simulink model "amr_integrated_delivery_system"  (R2025b)
settings: Solver=FixedStepDiscrete  StartTime=0.0  StopTime=90  FixedStep=0.05  RelTol=1e-3
settings Model: Creator=leeyj  LastModifiedBy=leeyj

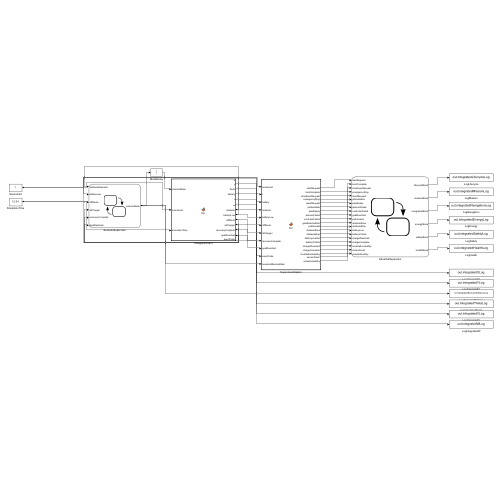
[thumbnail: Simulink's stored preview of the top-level diagram]
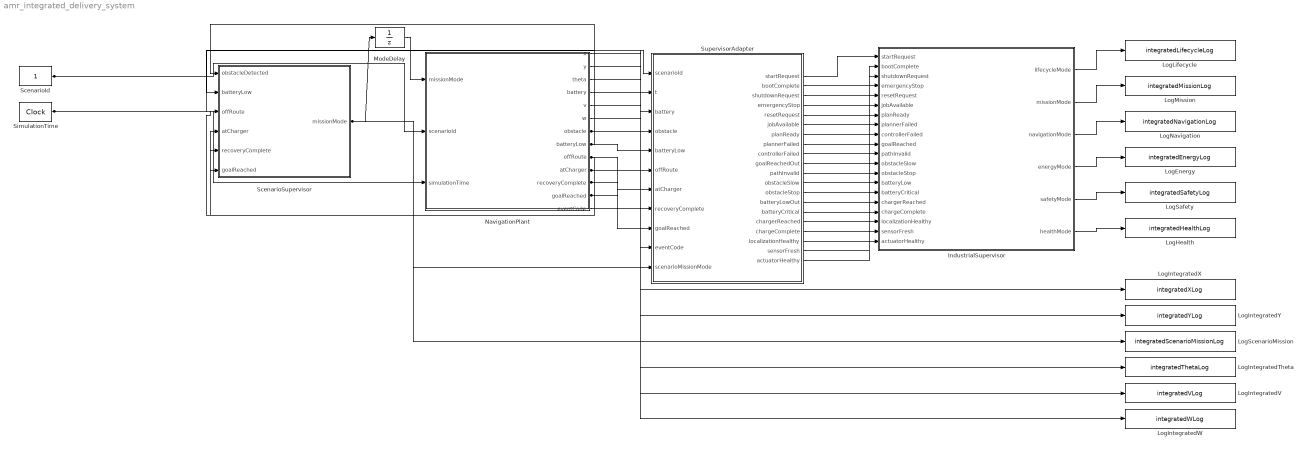
== system amr_integrated_delivery_system ==
  IndustrialSupervisor : Stateflow chart  TreatAsAtomicUnit=on
  LogEnergy : ToWorkspace  VariableName=integratedEnergyLog  SaveFormat=Timeseries  SampleTime=-1
  LogHealth : ToWorkspace  VariableName=integratedHealthLog  SaveFormat=Timeseries  SampleTime=-1
  LogIntegratedTheta : ToWorkspace  VariableName=integratedThetaLog  SaveFormat=Timeseries  SampleTime=-1
  LogIntegratedV : ToWorkspace  VariableName=integratedVLog  SaveFormat=Timeseries  SampleTime=-1
  LogIntegratedW : ToWorkspace  VariableName=integratedWLog  SaveFormat=Timeseries  SampleTime=-1
  LogIntegratedX : ToWorkspace  VariableName=integratedXLog  SaveFormat=Timeseries  SampleTime=-1
  LogIntegratedY : ToWorkspace  VariableName=integratedYLog  SaveFormat=Timeseries  SampleTime=-1
  LogLifecycle : ToWorkspace  VariableName=integratedLifecycleLog  SaveFormat=Timeseries  SampleTime=-1
  LogMission : ToWorkspace  VariableName=integratedMissionLog  SaveFormat=Timeseries  SampleTime=-1
  LogNavigation : ToWorkspace  VariableName=integratedNavigationLog  SaveFormat=Timeseries  SampleTime=-1
  LogSafety : ToWorkspace  VariableName=integratedSafetyLog  SaveFormat=Timeseries  SampleTime=-1
  LogScenarioMission : ToWorkspace  VariableName=integratedScenarioMissionLog  SaveFormat=Timeseries  SampleTime=-1
  ModeDelay : UnitDelay  SampleTime=0.05  HasFrameUpgradeWarning=on
  NavigationPlant : MATLAB Function  TreatAsAtomicUnit=on
  ScenarioId : Constant
  ScenarioSupervisor : Stateflow chart  TreatAsAtomicUnit=on
  SimulationTime : DigitalClock  SampleTime=0.05
  SupervisorAdapter : MATLAB Function  TreatAsAtomicUnit=on
  wires:
  ModeDelay/1 -> NavigationPlant/1(missionMode)
  ScenarioId/1 -> NavigationPlant/2(scenarioId), SupervisorAdapter/1(scenarioId)
  SimulationTime/1 -> NavigationPlant/3(simulationTime), SupervisorAdapter/2(t)
  NavigationPlant/7(obstacle) -> ScenarioSupervisor/1(obstacleDetected), SupervisorAdapter/4(obstacle)
  NavigationPlant/8(batteryLow) -> ScenarioSupervisor/2(batteryLow), SupervisorAdapter/5(batteryLow)
  NavigationPlant/9(offRoute) -> ScenarioSupervisor/3(offRoute), SupervisorAdapter/6(offRoute)
  NavigationPlant/10(atCharger) -> ScenarioSupervisor/4(atCharger), SupervisorAdapter/7(atCharger)
  NavigationPlant/11(recoveryComplete) -> ScenarioSupervisor/5(recoveryComplete), SupervisorAdapter/8(recoveryComplete)
  NavigationPlant/12(goalReached) -> ScenarioSupervisor/6(goalReached), SupervisorAdapter/9(goalReached)
  ScenarioSupervisor/1(missionMode) -> ModeDelay/1, SupervisorAdapter/11(scenarioMissionMode), LogScenarioMission/1
  NavigationPlant/4(battery) -> SupervisorAdapter/3(battery)
  NavigationPlant/13(eventCode) -> SupervisorAdapter/10(eventCode)
  SupervisorAdapter/1(startRequest) -> IndustrialSupervisor/1(startRequest)
  SupervisorAdapter/2(bootComplete) -> IndustrialSupervisor/2(bootComplete)
  SupervisorAdapter/3(shutdownRequest) -> IndustrialSupervisor/3(shutdownRequest)
  SupervisorAdapter/4(emergencyStop) -> IndustrialSupervisor/4(emergencyStop)
  SupervisorAdapter/5(resetRequest) -> IndustrialSupervisor/5(resetRequest)
  SupervisorAdapter/6(jobAvailable) -> IndustrialSupervisor/6(jobAvailable)
  SupervisorAdapter/7(planReady) -> IndustrialSupervisor/7(planReady)
  SupervisorAdapter/8(plannerFailed) -> IndustrialSupervisor/8(plannerFailed)
  SupervisorAdapter/9(controllerFailed) -> IndustrialSupervisor/9(controllerFailed)
  SupervisorAdapter/10(goalReachedOut) -> IndustrialSupervisor/10(goalReached)
  SupervisorAdapter/11(pathInvalid) -> IndustrialSupervisor/11(pathInvalid)
  SupervisorAdapter/12(obstacleSlow) -> IndustrialSupervisor/12(obstacleSlow)
  SupervisorAdapter/13(obstacleStop) -> IndustrialSupervisor/13(obstacleStop)
  SupervisorAdapter/14(batteryLowOut) -> IndustrialSupervisor/14(batteryLow)
  SupervisorAdapter/15(batteryCritical) -> IndustrialSupervisor/15(batteryCritical)
  SupervisorAdapter/16(chargerReached) -> IndustrialSupervisor/16(chargerReached)
  SupervisorAdapter/17(chargeComplete) -> IndustrialSupervisor/17(chargeComplete)
  SupervisorAdapter/18(localizationHealthy) -> IndustrialSupervisor/18(localizationHealthy)
  SupervisorAdapter/19(sensorFresh) -> IndustrialSupervisor/19(sensorFresh)
  SupervisorAdapter/20(actuatorHealthy) -> IndustrialSupervisor/20(actuatorHealthy)
  NavigationPlant/1(x) -> LogIntegratedX/1
  NavigationPlant/2(y) -> LogIntegratedY/1
  IndustrialSupervisor/1(lifecycleMode) -> LogLifecycle/1
  IndustrialSupervisor/2(missionMode) -> LogMission/1
  IndustrialSupervisor/3(navigationMode) -> LogNavigation/1
  IndustrialSupervisor/4(energyMode) -> LogEnergy/1
  IndustrialSupervisor/5(safetyMode) -> LogSafety/1
  IndustrialSupervisor/6(healthMode) -> LogHealth/1
  NavigationPlant/3(theta) -> LogIntegratedTheta/1
  NavigationPlant/5(v) -> LogIntegratedV/1
  NavigationPlant/6(w) -> LogIntegratedW/1

== stateflow chart amr_integrated_delivery_system/IndustrialSupervisor ==
  state Operational
    entry,during:
    lifecycleMode = uint8(2);
    state MissionRegion [parallel]
      settings: executionOrder=1
      state Idle
        entry,during:
        missionMode = uint8(0);
      state AcceptJob
        entry,during:
        missionMode = uint8(1);
      state NavigatePickup
        entry,during:
        missionMode = uint8(2);
      state Loading
        entry,during:
        missionMode = uint8(3);
      state NavigateDropoff
        entry,during:
        missionMode = uint8(4);
      state Unloading
        entry,during:
        missionMode = uint8(5);
      state ReturnHome
        entry,during:
        missionMode = uint8(6);
      (default) -> Idle
      Idle -> AcceptJob : [jobAvailable]
      ReturnHome -> Idle : [goalReached]
      AcceptJob -> NavigatePickup : after(0.5,sec)
      NavigatePickup -> Loading : [goalReached]
      Loading -> NavigateDropoff : after(1,sec)
      NavigateDropoff -> Unloading : [goalReached]
      Unloading -> ReturnHome : after(1,sec)
    state NavigationRegion [parallel]
      settings: executionOrder=2
      state NavIdle
        entry,during:
        navigationMode = uint8(0);
      state Planning
        entry,during:
        navigationMode = uint8(1);
      state Tracking
        entry,during:
        navigationMode = uint8(2);
      state Replanning
        entry,during:
        navigationMode = uint8(3);
      state Recovery
        entry,during:
        navigationMode = uint8(4);
      state NavFailed
        entry,during:
        navigationMode = uint8(5);
      (default) -> NavIdle
      Tracking -> NavIdle [order 3] : [goalReached]
      NavIdle -> Planning : [missionMode == uint8(2) || missionMode == uint8(4) || missionMode == uint8(6)]
      Planning -> Recovery [order 3] : after(3,sec)
      Planning -> Tracking [order 1] : [planReady]
      NavFailed -> Planning : [resetRequest]
      Recovery -> Planning [order 1] : [resetRequest]
      Planning -> Recovery [order 2] : [plannerFailed]
      Replanning -> Tracking [order 1] : [planReady]
      Tracking -> Recovery [order 2] : [controllerFailed]
      Tracking -> Replanning [order 1] : [pathInvalid]
      Replanning -> Recovery [order 2] : [plannerFailed]
      Replanning -> Recovery [order 3] : after(3,sec)
      Recovery -> NavFailed [order 2] : after(2,sec)
    state EnergyRegion [parallel]
      settings: executionOrder=3
      state EnergyNormal
        entry,during:
        energyMode = uint8(0);
      state EnergyLow
        entry,during:
        energyMode = uint8(1);
      state EnergyCritical
        entry,during:
        energyMode = uint8(2);
      state Charging
        entry,during:
        energyMode = uint8(3);
      (default) -> EnergyNormal
      EnergyLow -> EnergyNormal [order 1] : [~batteryLow]
      Charging -> EnergyNormal : [chargeComplete]
      EnergyNormal -> EnergyLow : [batteryLow]
      EnergyLow -> EnergyCritical [order 2] : [batteryCritical]
      EnergyCritical -> Charging : [chargerReached]
    state SafetyRegion [parallel]
      settings: executionOrder=4
      state Safe
        entry,during:
        safetyMode = uint8(0);
      state Slowdown
        entry,during:
        safetyMode = uint8(1);
      state ProtectiveStop
        entry,during:
        safetyMode = uint8(2);
      (default) -> Safe
      Safe -> Slowdown [order 1] : [obstacleSlow]
      ProtectiveStop -> Safe : [~obstacleStop && resetRequest]
      Safe -> ProtectiveStop [order 2] : [obstacleStop]
      Slowdown -> Safe [order 2] : [~obstacleSlow && ~obstacleStop]
      Slowdown -> ProtectiveStop [order 1] : [obstacleStop]
    state HealthRegion [parallel]
      settings: executionOrder=5
      state Healthy
        entry,during:
        healthMode = uint8(0);
      state Degraded
        entry,during:
        healthMode = uint8(1);
      state HealthFault
        entry,during:
        healthMode = uint8(2);
      (default) -> Healthy
      Healthy -> Degraded [order 1] : [~sensorFresh || ~localizationHealthy]
      Healthy -> HealthFault [order 2] : [~actuatorHealthy]
      Degraded -> Healthy [order 1] : [sensorFresh && localizationHealthy && actuatorHealthy]
      Degraded -> HealthFault [order 2] : [~actuatorHealthy]
      Degraded -> HealthFault [order 3] : after(5,sec)
  state PowerOff
    entry,during:
    lifecycleMode = uint8(0);
    missionMode = uint8(0);
    navigationMode = uint8(0);
    energyMode = uint8(0);
    safetyMode = uint8(0);
    healthMode = uint8(0);
  state Boot
    entry,during:
    lifecycleMode = uint8(1);
    missionMode = uint8(0);
    navigationMode = uint8(0);
    energyMode = uint8(0);
    safetyMode = uint8(0);
    healthMode = uint8(0);
  state ControlledShutdown
    entry,during:
    lifecycleMode = uint8(3);
    missionMode = uint8(0);
    navigationMode = uint8(0);
    energyMode = uint8(0);
    safetyMode = uint8(0);
    healthMode = uint8(0);
  state FaultLatched
    entry,during:
    lifecycleMode = uint8(4);
    missionMode = uint8(0);
    navigationMode = uint8(0);
    energyMode = uint8(0);
    safetyMode = uint8(3);
    healthMode = uint8(2);
  state EmergencyStopLatched
    entry,during:
    lifecycleMode = uint8(5);
    missionMode = uint8(0);
    navigationMode = uint8(0);
    energyMode = uint8(0);
    safetyMode = uint8(3);
    healthMode = uint8(2);
  (default) -> PowerOff
  ControlledShutdown -> PowerOff : after(1,sec)
  PowerOff -> Boot : [startRequest]
  Operational -> ControlledShutdown [order 1] : [shutdownRequest]
  FaultLatched -> Boot : [resetRequest && actuatorHealthy && sensorFresh]
  EmergencyStopLatched -> Boot : [resetRequest && ~emergencyStop]
  Boot -> Operational [order 1] : [bootComplete]
  Boot -> EmergencyStopLatched [order 2] : [emergencyStop]
  Operational -> FaultLatched [order 3] : [healthMode == uint8(2)]
  Operational -> EmergencyStopLatched [order 2] : [emergencyStop]
  data: startRequest input boolean size=1; bootComplete input boolean size=1; shutdownRequest input boolean size=1; emergencyStop input boolean size=1; resetRequest input boolean size=1; jobAvailable input boolean size=1; planReady input boolean size=1; plannerFailed input boolean size=1; controllerFailed input boolean size=1; goalReached input boolean size=1; pathInvalid input boolean size=1; obstacleSlow input boolean size=1; obstacleStop input boolean size=1; batteryLow input boolean size=1; batteryCritical input boolean size=1; chargerReached input boolean size=1; chargeComplete input boolean size=1; localizationHealthy input boolean size=1; sensorFresh input boolean size=1; actuatorHealthy input boolean size=1; lifecycleMode output uint8 size=1; missionMode output uint8 size=1; navigationMode output uint8 size=1; energyMode output uint8 size=1; safetyMode output uint8 size=1; healthMode output uint8 size=1

== matlab function amr_integrated_delivery_system/NavigationPlant ==
  data: x output double size=1; missionMode input uint8 size=1; y output double size=1; scenarioId input double size=1; simulationTime input double size=1; theta output double size=1; battery output double size=1; v output double size=1; w output double size=1; obstacle output boolean size=1; batteryLow output boolean size=1; offRoute output boolean size=1; atCharger output boolean size=1; recoveryComplete output boolean size=1; goalReached output boolean size=1; eventCode output uint8 size=1
function [x,y,theta,battery,v,w,obstacle,batteryLow,offRoute,atCharger,recoveryComplete,goalReached,eventCode] = fcn(missionMode,scenarioId,simulationTime)
coder.extrinsic('amr.scenarios.scenarioEngineStep');
x=0.0; y=0.0; theta=0.0; battery=0.0; v=0.0; w=0.0;
obstacle=false; batteryLow=false; offRoute=false; atCharger=false; recoveryComplete=false; goalReached=false; eventCode=uint8(0);
[x,y,theta,battery,v,w,obstacle,batteryLow,offRoute,atCharger,recoveryComplete,goalReached,eventCode] = amr.scenarios.scenarioEngineStep(uint8(missionMode),scenarioId,simulationTime);

== stateflow chart amr_integrated_delivery_system/ScenarioSupervisor ==
  state Rerouting
    entry,during:
    missionMode = uint8(7);
  state OffRouteStop
    entry,during:
    missionMode = uint8(6);
  state Initializing
    entry,during:
    missionMode = uint8(0);
  state Completed
    entry,during:
    missionMode = uint8(8);
  state Charging
    entry,during:
    missionMode = uint8(5);
  state Delivering
    entry,during:
    missionMode = uint8(1);
  state ReturnToCharger
    entry,during:
    missionMode = uint8(4);
  state ObstacleStop
    entry,during:
    missionMode = uint8(2);
  state AvoidingObstacle
    entry,during:
    missionMode = uint8(3);
  (default) -> Initializing
  OffRouteStop -> Rerouting : after(1,sec)
  Rerouting -> Delivering : [recoveryComplete]
  Delivering -> OffRouteStop [order 3] : [offRoute]
  Initializing -> Delivering : after(1,sec)
  Delivering -> Completed [order 4] : [goalReached]
  Delivering -> ObstacleStop [order 1] : [obstacleDetected]
  Charging -> Delivering : [recoveryComplete]
  AvoidingObstacle -> Delivering : [recoveryComplete]
  Delivering -> ReturnToCharger [order 2] : [batteryLow]
  ReturnToCharger -> Charging : [atCharger]
  ObstacleStop -> AvoidingObstacle : after(1,sec)
  data: obstacleDetected input boolean; batteryLow input boolean; offRoute input boolean; atCharger input boolean; recoveryComplete input boolean; goalReached input boolean; missionMode output uint8

== matlab function amr_integrated_delivery_system/SupervisorAdapter ==
  data: scenarioId input; startRequest output; t input; battery input; obstacle input; batteryLow input; offRoute input; atCharger input; recoveryComplete input; goalReached input; eventCode input; scenarioMissionMode input; bootComplete output; shutdownRequest output; emergencyStop output; resetRequest output; jobAvailable output; planReady output; plannerFailed output; controllerFailed output; goalReachedOut output; pathInvalid output; obstacleSlow output; obstacleStop output; batteryLowOut output; batteryCritical output; chargerReached output; chargeComplete output; localizationHealthy output; sensorFresh output; actuatorHealthy output
function [startRequest,bootComplete,shutdownRequest,emergencyStop,resetRequest,jobAvailable,planReady,plannerFailed,controllerFailed,goalReachedOut,pathInvalid,obstacleSlow,obstacleStop,batteryLowOut,batteryCritical,chargerReached,chargeComplete,localizationHealthy,sensorFresh,actuatorHealthy] = fcn(scenarioId,t,battery,obstacle,batteryLow,offRoute,atCharger,recoveryComplete,goalReached,eventCode,scenarioMissionMode)
startRequest = t >= 0.10 && scenarioMissionMode ~= uint8(8);
bootComplete = t >= 1.00;
shutdownRequest = scenarioMissionMode == uint8(8); emergencyStop = false;
resetRequest = recoveryComplete || (scenarioMissionMode == uint8(3) && ~obstacle) || scenarioMissionMode == uint8(7);
jobAvailable = t >= 1.20;
planReady = scenarioMissionMode == uint8(1) || scenarioMissionMode == uint8(3) || scenarioMissionMode == uint8(4) || scenarioMissionMode == uint8(7);
plannerFailed = false; controllerFailed = false;
goalReachedOut = goalReached; pathInvalid = obstacle || offRoute;
obstacleSlow = eventCode == uint8(6); obstacleStop = obstacle;
batteryLowOut = batteryLow; batteryCritical = battery <= 20.0;
chargerReached = atCharger;
chargeComplete = recoveryComplete && battery >= 89.0;
localizationHealthy = ~offRoute; sensorFresh = true; actuatorHealthy = true;
if scenarioId < 1, shutdownRequest = true; end
